simulink subsystem "Kinematics"  (R2022b)
settings: Solver=VariableStepAuto  StartTime=0.0  StopTime=10.0  RelTol=1e-3
undefined symbols (not defined in the file or in its folder): settings
libraries: simulink_extras x1
settings Model: Creator=Nicolò  LastModifiedBy=brent

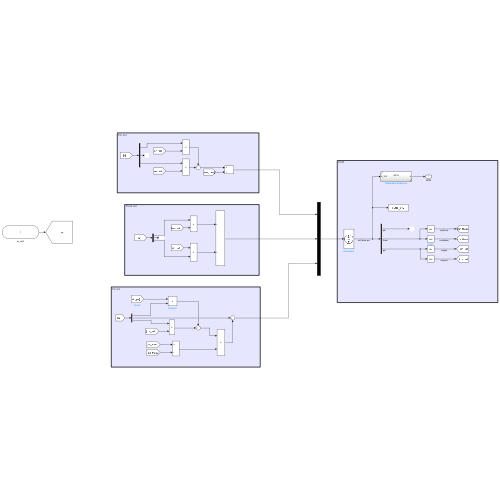
[thumbnail: Simulink's stored preview of the top-level diagram]
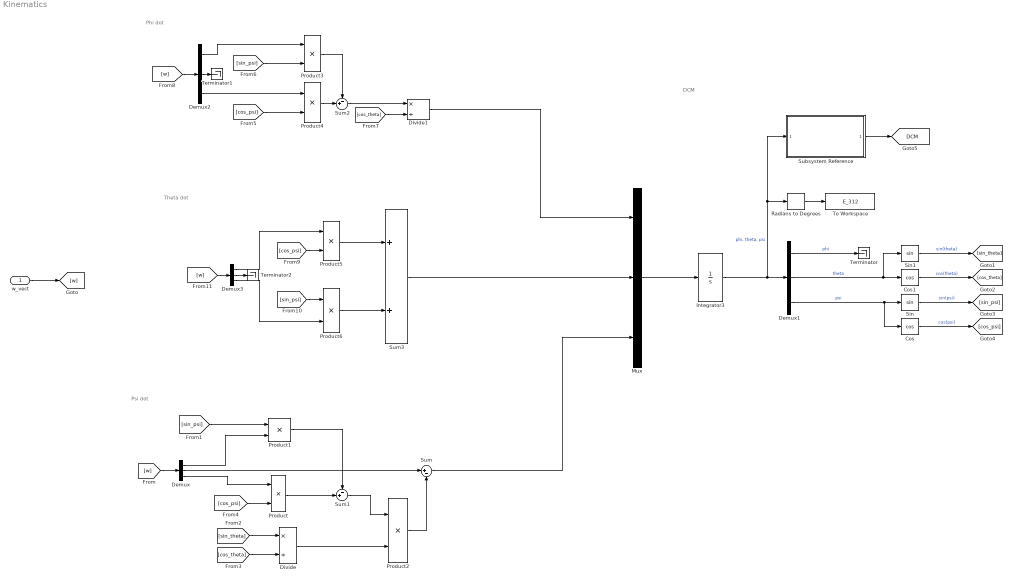
== system Kinematics ==
  note: DCM
  note: Theta dot
  note: Phi dot
  note: Psi dot
  w_vect : Inport
  Cos : Trigonometry  Operator=cos
  Cos1 : Trigonometry  Operator=cos
  Demux{,1..3} (4 alike) : Demux  Outputs=3
  Divide : Product  Inputs=*/
  Divide1 : Product  Inputs=*/
  Integrator3 : Integrator  InitialCondition=settings.E0  WrapState=on
  Mux : Mux  Inputs=3
  Product{,1..6} (7 alike) : Product
  Radians to Degrees : simulink_extras/Transformations/Radians to Degrees
  Sin : Trigonometry
  Sin1 : Trigonometry
  Subsystem Reference : Subsystem  ReferencedSubsystem=A312
  Sum : Sum  Inputs=|+-
  Sum1 : Sum  Inputs=-+|
  Sum2 : Sum  Inputs=-+|
  Sum3 : Sum
  Terminator : Terminator
  Terminator1 : Terminator
  Terminator2 : Terminator
  To Workspace : ToWorkspace  VariableName=E_312  SampleTime=-1
  tag scope: DCM=global
  wires:
  Integrator3/1 -> Subsystem Reference/1, Radians to Degrees/1, Demux1/1  "phi, theta, psi"
  w_vect/1 -> [w]
  Demux1/1 -> Terminator/1  "phi"
  Sin1/1 -> [sin_theta]  "sin(theta)"
  Cos1/1 -> [cos_theta]  "cos(theta)"
  Cos/1 -> [cos_psi]  "cos(psi)"
  Demux1/3 -> Cos/1, Sin/1  "psi"
  Sin/1 -> [sin_psi]  "sin(psi)"
  Demux1/2 -> Sin1/1, Cos1/1  "theta"
  Demux/2 -> Sum/1
  [sin_theta] -> Divide/1
  [sin_psi] -> Product1/1
  [cos_theta] -> Divide/2
  Demux/3 -> Product/1
  Product2/1 -> Sum/2
  [cos_psi] -> Product/2
  Demux/1 -> Product1/2
  Sum/1 -> Mux/3
  Divide/1 -> Product2/2
  Sum1/1 -> Product2/1
  Product/1 -> Sum1/2
  Product1/1 -> Sum1/1
  [w] -> Demux/1
  Divide1/1 -> Mux/1
  Sum2/1 -> Divide1/1
  Product4/1 -> Sum2/2
  [cos_theta] -> Divide1/2
  Demux2/3 -> Product4/1
  [sin_psi] -> Product3/2
  [cos_psi] -> Product4/2
  Product3/1 -> Sum2/1
  Demux2/1 -> Product3/1
  [w] -> Demux2/1
  Demux2/2 -> Terminator1/1
  Product5/1 -> Sum3/1
  Sum3/1 -> Mux/2
  Product6/1 -> Sum3/2
  [w] -> Demux3/1
  Demux3/1 -> Product5/1
  [cos_psi] -> Product5/2
  Demux3/3 -> Product6/2
  [sin_psi] -> Product6/1
  Demux3/2 -> Terminator2/1
  Mux/1 -> Integrator3/1
  Subsystem Reference/1 -> [DCM]
  Radians to Degrees/1 -> To Workspace/1
